simulink model "LeftArmAgent"  (Simulink 6.5)
settings: Solver=ode45  SolverMode=SingleTasking  StartTime=0.0  StopTime=10.0  RelTol=1e-3  AbsTol=1e-6
settings Model: Creator=The MathWorks Inc.  LastModifiedBy=suarezjl  ExtModeTrigMode=oneshot  ExtModeArmWhenConnect=off  ExtModeAutoUpdateStatusClock=off
settings DataIOCC: LimitDataPoints=off  SignalLoggingName=logsOut
settings OptimizationCC: BooleanDataType=off  InlineInvariantSignals=on
settings DebuggingCC: CheckExecutionContextPreStartOutputMsg=on  CheckExecutionContextRuntimeOutputMsg=on  SolverPrmCheckMsg=none  MultiTaskDSMMsg=warning  MultiTaskCondExecSysMsg=none  IntegerOverflowMsg=none  StrictBusMsg=None
settings HardwareCC: TargetUnknown=on
settings ModelReferenceCC: UpdateModelReferenceTargets=IfOutOfDate
settings RTWCC: IncludeERTFirstTime=on

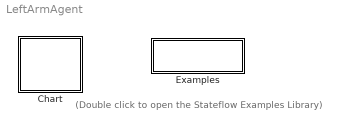
== system LeftArmAgent ==
  note: (Double click to open the
      | Stateflow Examples Library)
  Chart : Stateflow chart
  Examples : Subsystem
      settings: OpenFcn=sf('Private','sf_examples')
      mask Display: disp('Examples')

== system LeftArmAgent/Examples ==

== stateflow chart Chart ==
  state InitialArmRoutine
    HungerForce\LeftArm\HomingController.ComputeHomingPressures()
    HungerForce\LeftArm\SampleIndPressure.HW_IO_6()
    HungerForce\LeftArm\StateMachine.Wait(50)
  state InitializeFunctions
    HungerForce\LeftArm\HomingController.Initial()
    HungerForce\LeftArm\SampleIndPressure.Initialize()
    HungerForce\LeftArm\PIDNonLinCtrl.Initial()
    HungerForce\LeftArm\ForwardKinematics.Initialize()
    HungerForce\LeftArm\InverseKinematics.Initialize()
    HungerForce\LeftArm\SampleIndPressure.Disable_ZMasking()
  state WriteHomeDesiredLogicalAngles
    HungerForce\LeftArm\SampleIndPressure.Enable_ZMasking()
    HungerForce\LeftArm\SampleIndPressure.WriteHomePositions()
  state LoadHomePosition
    HungerForce\LeftArm\SampleIndPressure.HW_IO_6()
    HungerForce\LeftArm\PIDNonLinCtrl.PID_NonLin_6Press()
    HungerForce\LeftArm\ForwardKinematics.ForwardKinematics()
    HungerForce\LeftArm\InverseKinematics.InverseKinematics()
  state PID_NonLinCtrlLoop
    HungerForce\LeftArm\Filter.FilterDesiredAngles()
    HungerForce\LeftArm\PIDNonLinCtrl.PID_NonLin_12Press()
    HungerForce\LeftArm\SampleIndPressure.HW_IO_12()
    HungerForce\LeftArm\PIDNonLinCtrl.Read_CurrentPressure()
    HungerForce\LeftArm\ForwardKinematics.ForwardKinematics()
    HungerForce\LeftArm\InverseKinematics.InverseKinematics()
    HungerForce\LeftArm\StateMachine.Wait(50)
  state Stop
    HungerForce\RightArm\SampleIndPressure.Reset()
  (default) -> InitializeFunctions : Start
  InitialArmRoutine -> InitialArmRoutine [order 1] : Default
  InitializeFunctions -> InitialArmRoutine : Always
  WriteHomeDesiredLogicalAngles -> LoadHomePosition : Always
  LoadHomePosition -> PID_NonLinCtrlLoop : Always
  InitialArmRoutine -> WriteHomeDesiredLogicalAngles [order 2] : Signal="Go to next state"
  PID_NonLinCtrlLoop -> PID_NonLinCtrlLoop [order 1] : Default
  PID_NonLinCtrlLoop -> Stop [order 2] : Signal="Stop"
